simulink model "cont_PI10V_31250f_v3"  (R2018a)
settings: Solver=VariableStepAuto  StartTime=0.0  StopTime=0.2  MaxStep=1e-4  RelTol=1e-4  EnableMultiTasking=on
libraries: powerlib x24, pePowerMeasurement x2, simulink x1, powerlib_meascontrol x1
Description:
  | Copyright 2008-2018 The MathWorks, Inc.
settings Model: Creator=MathWorks  LastModifiedBy=Batu
settings SolverCC: SolverResetMethod=Robust
settings DataIOCC: ReturnWorkspaceOutputs=on
settings OptimizationCC: LifeSpan=inf
settings DebuggingCC: ReadBeforeWriteMsg=DisableAll  WriteAfterWriteMsg=DisableAll  WriteAfterReadMsg=DisableAll  MultiTaskDSMMsg=none  SFUnexpectedBacktrackingDiag=warning  SFNoUnconditionalDefaultTransitionDiag=warning  SFExecutionAtInitializationDiag=none
settings ModelReferenceCC: UpdateModelReferenceTargets=IfOutOfDate
settings SFSimCC: SFSimEcho=off
settings CodeAppCC: StateflowObjectComments=on
settings GRTTargetCC: TargetLangStandard=C89/C90 (ANSI)  GeneratePreprocessorConditionals=Disable all
settings ConfigComp: CovMetricSettings=dw  CovHtmlReporting=on  CovSaveCumulativeToWorkspaceVar=on  CovSaveSingleToWorkspaceVar=on  CovExternalEMLEnable=off
settings SimscapeCC: SimscapeNormalizeSystem=off  SimscapeNominalValues={1, 'bar'; 1, 'cm^3/s'; 1, 'bar*kg/s'; 1, 'kJ/kg'; 1, 'kW'; }

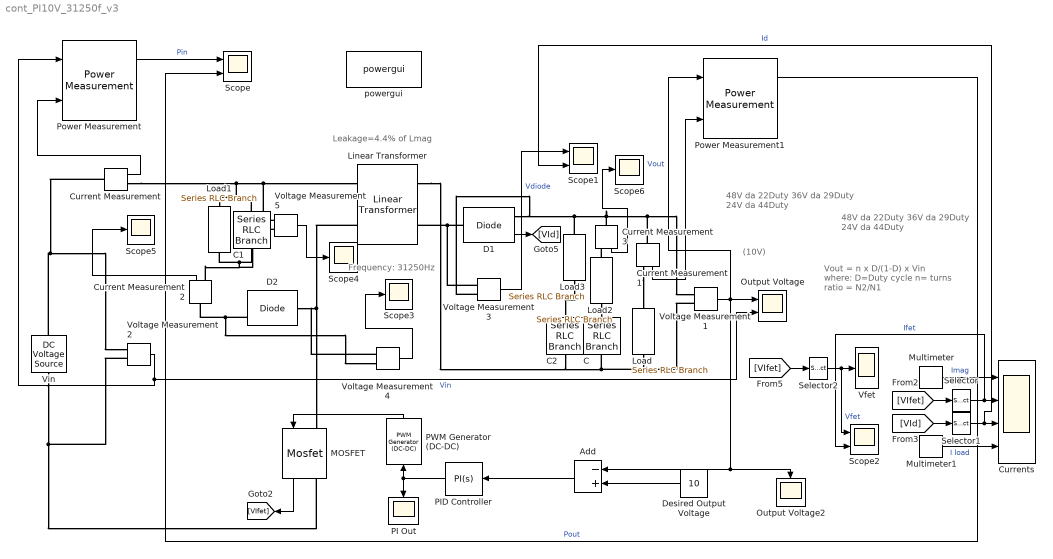
== system cont_PI10V_31250f_v3 ==
  note: Frequency: 31250Hz
  note: (10V)
  note: Leakage=4.4% of Lmag
  note: Vout = n x D/(1-D) x Vin
      | where: D=Duty cycle
      | n= turns ratio = N2/N1
  note: 48V da 22Duty
      | 36V da 29Duty
      | 24V da 44Duty
  note: 48V da 22Duty
      | 36V da 29Duty
      | 24V da 44Duty
  Add : Sum  Inputs=-+
  C : powerlib/Elements/Series RLC Branch  LConnTagsString=__new0  RConnTagsString=__new0  BranchType=C  Resistance=1e-4  Inductance=200e-6  SetiL0=off  InitialCurrent=0  Capacitance=330e-6  Setx0=off  InitialVoltage=0  Measurements=None
  C1 : powerlib/Elements/Series RLC Branch  LConnTagsString=__new0  RConnTagsString=__new0  BranchType=C  Resistance=1e-4  Inductance=200e-6  SetiL0=off  InitialCurrent=0  Capacitance=0.022e-6  Setx0=off  InitialVoltage=0  Measurements=None
  C2 : powerlib/Elements/Series RLC Branch  LConnTagsString=__new0  RConnTagsString=__new0  BranchType=C  Resistance=1e-4  Inductance=200e-6  SetiL0=off  InitialCurrent=0  Capacitance=330e-6  Setx0=off  InitialVoltage=0  Measurements=None
  Current Measurement{,1..3} (4 alike) : powerlib/Measurements/Current Measurement  PhasorSimulation=off  OutputType=Complex  PSBequivalent=0
  Currents : Scope  NumInputPorts=4
  D1 : powerlib/Power Electronics/Diode  Ron=1e-3  Lon=0  Vf=0.8  IC=0  UseSnubber=off  Rs=inf  Cs=0  Measurements=on
  D2 : powerlib/Power Electronics/Diode  Ron=1e-3  Lon=0  Vf=0.8  IC=0  UseSnubber=off  Rs=inf  Cs=0  Measurements=on
  Desired Output Voltage : Constant  Value=10
  Linear Transformer : powerlib/Elements/Linear Transformer  UNITS=SI  NominalPower=[ 90 31370 ]  winding1=[34 0.07 1.3e-6]  winding2=[20 0 0]  ThreeWindings=off  winding3=[3.15e+05 3.969e+07 6316.9]  RmLm=[1e4 26e-6]  Measurements=Magnetization current  DataType=on
  Load : powerlib/Elements/Series RLC Branch  LConnTagsString=__new0  RConnTagsString=__new0  BranchType=R  Resistance=1.67  Inductance=200e-6  SetiL0=off  InitialCurrent=0  Capacitance=400e-6  Setx0=off  InitialVoltage=0  Measurements=Branch current
  Load1 : powerlib/Elements/Series RLC Branch  LConnTagsString=__new0  RConnTagsString=__new0  BranchType=R  Resistance=22e1  Inductance=200e-6  SetiL0=off  InitialCurrent=0  Capacitance=400e-6  Setx0=off  InitialVoltage=0  Measurements=Branch current
  Load2 : powerlib/Elements/Series RLC Branch  LConnTagsString=__new0  RConnTagsString=__new0  BranchType=R  Resistance=0.1  Inductance=200e-6  SetiL0=off  InitialCurrent=0  Capacitance=400e-6  Setx0=off  InitialVoltage=0  Measurements=Branch current
  Load3 : powerlib/Elements/Series RLC Branch  LConnTagsString=__new0  RConnTagsString=__new0  BranchType=R  Resistance=0.005  Inductance=200e-6  SetiL0=off  InitialCurrent=0  Capacitance=400e-6  Setx0=off  InitialVoltage=0  Measurements=Branch current
  MOSFET : powerlib/Power Electronics/Mosfet  Ron=1e-3  Lon=0  Rd=1e-3  Vfd=0.5  IC=0  Rs=1e9  Cs=inf  Measurements=on
  Multimeter : powerlib/Measurements/Multimeter  PhasorSimulation=off  OutputType=Complex  sel=6  L=7  Gain=1  yselected={'Imag: Linear Transformer'};  PSBOutputType=1  PSBequivalent=0  AxesSetting=[0,0.1,-100,100]  Display=0  SavedBlockNames=-11
  Multimeter1 : powerlib/Measurements/Multimeter  PhasorSimulation=off  OutputType=Complex  sel=1  L=7  Gain=1  yselected={'Ib: Load'};  PSBOutputType=1  PSBequivalent=0  AxesSetting=[0,0.1,-100,100]  Display=0  SavedBlockNames=-11
  Output Voltage : Scope  NumInputPorts=2
  Output Voltage2 : Scope
  PI Out : Scope
  PID Controller : simulink/Continuous/PID Controller  Controller=PI  TimeDomain=Continuous-time  SampleTime=-1  IntegratorMethod=Forward Euler  FilterMethod=Forward Euler  Form=Parallel  UseFilter=on  ControllerParametersSource=internal  P=0.04  I=10  D=0  N=100  InitialConditionSource=internal  InitialConditionForIntegrator=0  InitialConditionForFilter=0  ExternalReset=none  LimitOutput=off  UpperSaturationLimit=inf  LowerSaturationLimit=-inf  LinearizeAsGain=on  AntiWindupMode=none  Kb=1  TrackingMode=off  Kt=1  PParamMin=[]  PParamMax=[]  IParamMin=[]  IParamMax=[]  DParamMin=[]  DParamMax=[]  NParamMin=[]  NParamMax=[]  KbParamMin=[]  KbParamMax=[]  KtParamMin=[]  KtParamMax=[]  POutMin=[]  POutMax=[]  IOutMin=[]  IOutMax=[]  DOutMin=[]  DOutMax=[]  NOutMin=[]  NOutMax=[]  KbOutMin=[]  KbOutMax=[]  KtOutMin=[]  KtOutMax=[]  IntegratorOutMin=[]  IntegratorOutMax=[]  FilterOutMin=[]  FilterOutMax=[]  SumOutMin=[]  SumOutMax=[]  SumI1OutMin=[]  SumI1OutMax=[]  SumI2OutMin=[]  SumI2OutMax=[]  SumI3OutMin=[]  SumI3OutMax=[]  SumDOutMin=[]  SumDOutMax=[]  SaturationOutMin=[]  SaturationOutMax=[]  IntegratorContinuousStateAttributes=''  IntegratorStateMustResolveToSignalObject=off  IntegratorRTWStateStorageClass=Auto  FilterContinuousStateAttributes=''  FilterStateMustResolveToSignalObject=off  FilterRTWStateStorageClass=Auto  DifferentiatorICPrevScaledInput=0  DifferentiatorOutMin=[]  DifferentiatorOutMax=[]  InitialConditionSetting=State (most efficient)  FilterDiffOutCoefMin=[]  FilterDiffOutCoefMax=[]  SumDenOutMin=[]  SumDenOutMax=[]  SumNumOutMin=[]  SumNumOutMax=[]  ReciprocalOutMin=[]  ReciprocalOutMax=[]  DivideOutMin=[]  DivideOutMax=[]  TunerSelectOption=Transfer Function Based (PID Tuner App)
  PWM Generator (DC-DC) : powerlib_meascontrol/Pulse & Signal Generators/PWM Generator (DC-DC)  Fsw=31370  Ts=0
  Power Measurement : pePowerMeasurement/Power Measurement  OverrideUsingVariant=Continuous  F=60  K=[0 1 2 3]  Ts=0
  Power Measurement1 : pePowerMeasurement/Power Measurement  OverrideUsingVariant=Continuous  F=60  K=[0 1 2 3]  Ts=0
  Scope : Scope  NumInputPorts=2
  Scope1 : Scope  NumInputPorts=2
  Scope2 : Scope  NumInputPorts=2
  Scope{3..6} (4 alike) : Scope
  Selector : Selector  InputPortWidth=2  IndexOptions=Index vector (dialog)  Indices=1  OutputSizes=1
  Selector1 : Selector  InputPortWidth=2  IndexOptions=Index vector (dialog)  Indices=1  OutputSizes=1
  Selector2 : Selector  InputPortWidth=2  IndexOptions=Index vector (dialog)  Indices=2  OutputSizes=1
  Vfet : Scope
  Vin : powerlib/Electrical Sources/DC Voltage Source  Amplitude=24  Measurements=None
  Voltage Measurement{1..5} (5 alike) : powerlib/Measurements/Voltage Measurement  PhasorSimulation=off  OutputType=Complex  PSBequivalent=0
  powergui : powerlib/powergui  Priority=1  SimulationMode=Continuous  SampleTime=50e-6  frequency=60  Iterations=50  frequencyindice=0  Pbase=100e6  ErrMax=1e-4  UnitsV=kV  UnitsW=MW  buscounter=0  FunctionMessages=off  echomessages=off  EnableUseOfTLC=off  CurrentSourceSwitches=off  DisableSnubberDevices=off  DisableRonSwitches=off  DisableVfSwitches=off  DisplayEquations=off  SolverType=Tustin/Backward Euler (TBE)  Interpol=off  ExternalGateDelay=off  methode=off  Ts=100  x0status=blocks  SPID=on  SwTol=0  HookPort=off  RestoreLinks=warning  ResistiveCurrentMeasurement=off  Frange=[0:2:500]  Ylog=off  Xlog=on  ShowGrid=off  save=off  variable=ZData  structure=0  ZoomFFT=off  StartTime=0.0  cycles=1  DisplayStyle=1  fundamental=60  FreqAxis=off  MaxFrequency=1000  frequencyindicesteady=1  RmsSteady=1  display=off
  wires:
  MOSFET/1 -> [VIfet]
  D1/1 -> [VId]
  Multimeter/1 -> Currents/1  "Imag"
  Selector/1 -> Scope2/2, Currents/2  "Ifet"
  [VIfet] -> Selector/1
  Selector1/1 -> Scope1/2, Currents/3  "Id"
  [VId] -> Selector1/1
  Multimeter1/1 -> Currents/4  "I load"
  Selector2/1 -> Scope2/1, Vfet/1  "Vfet"
  [VIfet] -> Selector2/1
  Add/1 -> PID Controller/1
  PID Controller/1 -> PI Out/1, PWM Generator (DC-DC)/1
  Desired Output Voltage/1 -> Add/2
  Voltage Measurement1/1 -> Output Voltage/1, Power Measurement1/1, Output Voltage2/1, Add/1  "Vout"
  Voltage Measurement2/1 -> Power Measurement/1, Output Voltage/2  "Vin"
  Current Measurement/1 -> Power Measurement/2
  Power Measurement/1 -> Scope/1  "Pin"
  Current Measurement1/1 -> Power Measurement1/2
  Power Measurement1/1 -> Scope/2  "Pout"
  Voltage Measurement3/1 -> Scope1/1  "Vdiode"
  PWM Generator (DC-DC)/1 -> MOSFET/1
  Voltage Measurement4/1 -> Scope3/1
  Voltage Measurement5/1 -> Scope4/1
  Current Measurement2/1 -> Scope5/1
  Current Measurement3/1 -> Scope6/1
  connections:
  Voltage Measurement3/LConn2 -- D1/RConn1 -- Load3/LConn1 -- Current Measurement3/LConn1 -- Current Measurement1/LConn1 -- Voltage Measurement1/LConn1
  Load/RConn1 -- Linear Transformer/RConn1 -- C2/RConn1 -- C/RConn1 -- Voltage Measurement1/LConn2
  Linear Transformer/LConn2 -- Voltage Measurement4/LConn1 -- D2/LConn1 -- MOSFET/LConn1
  D1/LConn1 -- Voltage Measurement3/LConn1 -- Linear Transformer/RConn2
  Vin/LConn1 -- Voltage Measurement2/LConn2 -- MOSFET/RConn1
  Vin/RConn1 -- Current Measurement/LConn1 -- Voltage Measurement2/LConn1
  C1/RConn1 -- Current Measurement2/RConn1 -- Voltage Measurement5/LConn2 -- Load1/RConn1
  C1/LConn1 -- Voltage Measurement5/LConn1 -- Linear Transformer/LConn1 -- Current Measurement/RConn1 -- Load1/LConn1
  Current Measurement1/RConn1 -- Load/LConn1
  D2/RConn1 -- Current Measurement2/LConn1 -- Voltage Measurement4/LConn2
  Load2/LConn1 -- Current Measurement3/RConn1
  Load2/RConn1 -- C/LConn1
  Load3/RConn1 -- C2/LConn1
